simulink model "simpleHelicopter_reference"  (R2023a)
settings: Solver=FixedStepAuto  StartTime=0.0  StopTime=500  FixedStep=fixedStepSize  RelTol=1e-3
model workspace: external: MATLAB File .\turboShaftEngine\initialization.m (data not in the file)
libraries: simulink x2, fl_lib x1, nesl_utility x1
settings Model: Creator=imyrsini  LastModifiedBy=imyrsini
settings HardwareCC: ProdBitPerLong=64  ProdHWDeviceType=Intel->x86-64 (Linux 64)
settings RTWCC: Description=Simulink Desktop Real-Time  SystemTargetFile=sldrt.tlc  TemplateMakefile=sldrt.tmf  RTWCompilerOptimization=on
settings CodeAppCC: MaxIdLength=95
settings SimulinkDesktopRealTimeCC: TargetLibSuffix=_sldrt.a  TargetPreCompLibLocation=L:\ML_MATLAB64\R2023a\toolbox\sldrt\lib\win64
settings SimscapeCC: SimscapeLogType=all  SimscapeLogSimulationStatistics=on  SimscapeLogToSDI=on

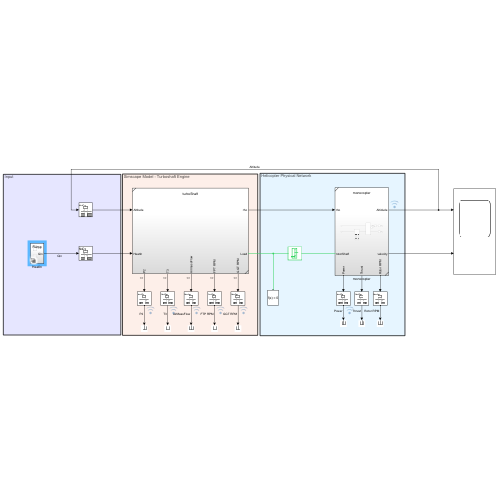
[thumbnail: Simulink's stored preview of the top-level diagram]
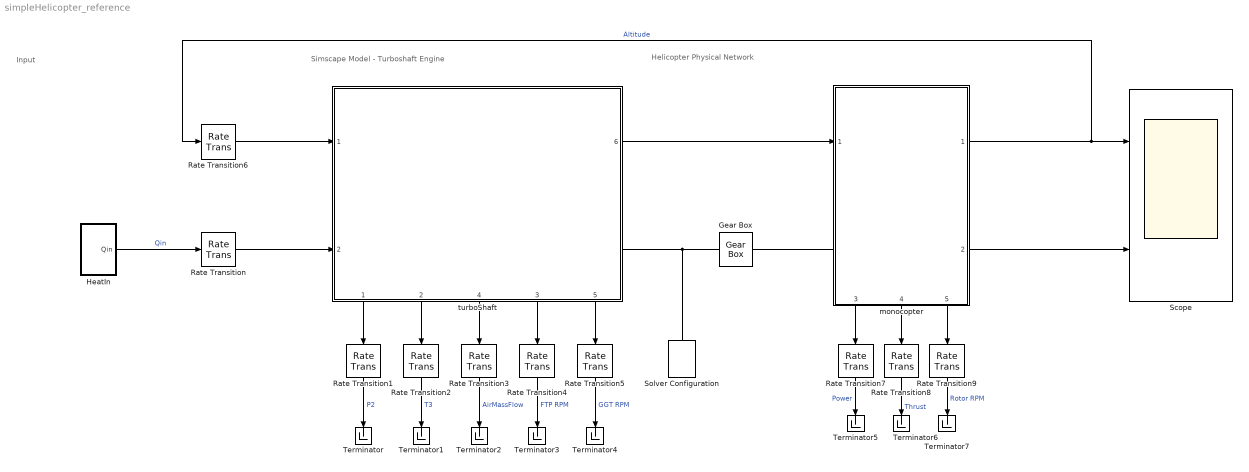
== system simpleHelicopter_reference ==
  note: Helicopter Physical Network
  note: Input
  note: Simscape Model - Turboshaft Engine
  Gear Box : fl_lib/Mechanical/Mechanisms/Gear Box  ratio=shaftFTP.GearRatio  t_in_specify=off  t_in_priority=None  t_in=0 N*m  t_in_nominal_specify=off  t_in_nominal_unit=N*m  t_in_nominal_value=1  t_out_specify=off  t_out_priority=None  t_out=0 N*m  t_out_nominal_specify=off  t_out_nominal_unit=N*m  t_out_nominal_value=1
  HeatIn : Subsystem  Variant=on  VariantControlMode=label  VariantControl=Choice  LabelModeActiveChoice=Ramp
  Rate Transition{,1..9} (10 alike) : RateTransition
  Scope : Scope  NumInputPorts=2
  Solver Configuration : nesl_utility/Solver Configuration  PhysicalDomain=network_engine_domain  SubClassName=solver  LeftPortType=input  RightPortType=generic  Tones=[]  Harmonics=[]  SimulateNoise=off  Profile=off  UseLocalSampling=off  EnableSwitchedLinearOptims=on  FrequencyDomain=off  UseCCode=off  RelTol=0.001  AbsTol=0.001  MinStep=1e-09  ToWorkspace=off  RevertToSquareIcSolve=off  NumHomotopyIterations=100  PhasorMode=off  PhasorModeNumHarmonics=1  ConsistencySolver=NEWTON_XTOL_AFTER_FTOL  IndexReductionMethod=DerivativeReplacement  DoDC=on  ResidualTolerance=1e-09  ConsistencyTolSource=GLOBAL  ConsistencyAbsTol=0.001  ConsistencyRelTol=0.001  ConsistencyTolFactor=0.001  UseLocalSolver=off  LocalSolverChoice=NE_BACKWARD_EULER_ADVANCER  ResolveIndetEquations=on  FunctionEvalNumThread=1  LocalSolverSampleTime=0.001  DoFixedCost=off  MaxNonlinIter=3  MaxModeIter=2  ComputeImpulses=off  ImpulseIterations=2  LinearAlgebra=auto  LinearAlgebraNumThread=0  EquationFormulation=NE_TIME_EF  DelaysMemoryBudget=1024  AutomaticFiltering=on  FilteringTimeConstant=0.001  PartitionStorageMethod=AS_NEEDED  PartitionMemoryBudget=1024  PartitionMethod=ROBUST
  Terminator{,1..7} (8 alike) : Terminator
  monocopter : Subsystem  ReferencedSubsystem=monocopter
      settings: PortSchema="{\"entries\":[{\"content\":{\"sides\":[{\"content\":{\"connectorIds\":[\"In1\",\"LConn1\"]},\"type\":\"ConnectorPlacement.EquallySpacedRectSide\",\"uuid\":\"2ecbf831-8a46-4c85-bf63-980a752dd5b1\"},{\"content\":{\"connectorIds\":[\"Out1\",\"Out2\"],\"side\":\"RIGHT\"},\"type\":\"ConnectorPlacement.EquallySpacedRectSide\",\"uuid\":\"e1b9456e-2a06-4a0b-bd2d-ca850f525143\"},{\"content\":{\"side\":\"TOP\"},\"type\":\"ConnectorPlacement.EquallySpacedRectSide\",\"uuid\":\"495d5151-b094-4c59-ad95-48151a95ddaf\"},{\"content\":{\"connectorIds\":[\"Out3\",\"Out4\",\"Out5\"],\"side\":\"BOTTOM\"},\"type\":\"ConnectorPlacement.EquallySpacedRectSide\",\"uuid\":\"d711d358-7c2d-4243-addb-9f7f6c9821dd\"}]},\"type\":\"ConnectorPlacement.EquallySpacedConnector\",\"uuid\":\"3949e89b-de6d-4024-bd06-1eddfa87edaa\"}],\"packageUris\":[\"http://schema.mathworks.com/mf0/Connector/R2020b\"],\"version\":\"1.0\"}"
  turboShaft : Subsystem  ReferencedSubsystem=turboShaft
      settings: PortSchema="{\"entries\":[{\"content\":{\"sides\":[{\"content\":{\"connectorIds\":[\"In1\",\"In2\"]},\"type\":\"ConnectorPlacement.EquallySpacedRectSide\",\"uuid\":\"7ef2fcb2-1b0d-44c2-984d-f1d7df0d7e80\"},{\"content\":{\"connectorIds\":[\"Out6\",\"RConn1\"],\"side\":\"RIGHT\"},\"type\":\"ConnectorPlacement.EquallySpacedRectSide\",\"uuid\":\"b2d8a67b-1c6d-4b5e-865c-86345858511b\"},{\"content\":{\"side\":\"TOP\"},\"type\":\"ConnectorPlacement.EquallySpacedRectSide\",\"uuid\":\"4c7a9b07-6c1b-4859-8cda-a5c2cd89c129\"},{\"content\":{\"connectorIds\":[\"Out1\",\"Out2\",\"Out4\",\"Out3\",\"Out5\"],\"side\":\"BOTTOM\"},\"type\":\"ConnectorPlacement.EquallySpacedRectSide\",\"uuid\":\"794a4e7c-d3e7-4ff8-9cf4-b7022afdc3bd\"}]},\"type\":\"ConnectorPlacement.EquallySpacedConnector\",\"uuid\":\"5f81fd46-9bac-4f96-9ad1-c3a7cd36c01a\"}],\"packageUris\":[\"http://schema.mathworks.com/mf0/Connector/R2020b\"],\"version\":\"1.0\"}"
  wires:
  HeatIn/1(Qin) -> Rate Transition/1  "Qin"
  turboShaft/1 -> Rate Transition1/1
  turboShaft/2 -> Rate Transition2/1
  turboShaft/4 -> Rate Transition3/1
  turboShaft/3 -> Rate Transition4/1
  turboShaft/5 -> Rate Transition5/1
  Rate Transition/1 -> turboShaft/2
  turboShaft/6 -> monocopter/1
  monocopter/2 -> Scope/2
  monocopter/3 -> Rate Transition7/1
  monocopter/4 -> Rate Transition8/1
  monocopter/5 -> Rate Transition9/1
  Rate Transition1/1 -> Terminator/1  "P2"
  Rate Transition2/1 -> Terminator1/1  "T3"
  Rate Transition3/1 -> Terminator2/1  "AirMassFlow"
  Rate Transition4/1 -> Terminator3/1  "FTP RPM"
  Rate Transition5/1 -> Terminator4/1  "GGT RPM"
  Rate Transition6/1 -> turboShaft/1
  Rate Transition7/1 -> Terminator5/1  "Power"
  Rate Transition8/1 -> Terminator6/1  "Thrust"
  Rate Transition9/1 -> Terminator7/1  "Rotor RPM"
  monocopter/1 -> Rate Transition6/1, Scope/1  "Altitude"
  connections:
  turboShaft/RConn1 -- Gear Box/LConn1 -- Solver Configuration/RConn1
  Gear Box/RConn1 -- monocopter/LConn1

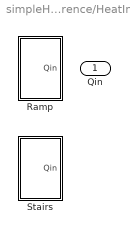
== system simpleHelicopter_reference/HeatIn ==
  Ramp : Subsystem  VariantControl=Ramp
  Stairs : Subsystem  VariantControl=Stairs
  Qin : Outport

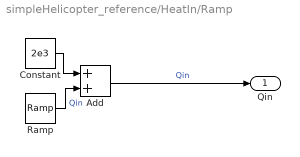
== system simpleHelicopter_reference/HeatIn/Ramp ==
  Add : Sum
  Constant : Constant  Value=2e3
  Ramp : simulink/Sources/Ramp  slope=6  start=10  InitialOutput=0
  Qin : Outport
  wires:
  Ramp/1 -> Add/2  "Qin"
  Constant/1 -> Add/1
  Add/1 -> Qin/1  "Qin"

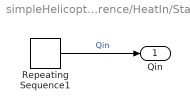
== system simpleHelicopter_reference/HeatIn/Stairs ==
  Repeating Sequence1 : simulink/Sources/Repeating Sequence  rep_seq_t=Qin_time  rep_seq_y=Qin
  Qin : Outport
  wires:
  Repeating Sequence1/1 -> Qin/1  "Qin"
